simulink model "massbalancer3"  (R2024a)
settings: Solver=ode45  StartTime=0.0  StopTime=300  MaxStep=0.5  RelTol=1e-3
libraries: matrix_library x29, sharedutil x3, sharedtransform x2, dspinverses x1, aerolibutil x1
(part 3 of 3)

== system massbalancer3/TNet/TBalances/Term2/Subsystem1 ==
  R_0 : Inport
  Reshape : Reshape  OutputDimensionality=Column vector (2-D)  OutputDimensions=[1,3]
  Selector : Selector  InputPortWidth=9  IndexOptions=Index vector (dialog)  Indices=[1]  OutputSizes=1
  Selector1 : Selector  InputPortWidth=9  IndexOptions=Index vector (dialog)  Indices=[2]  OutputSizes=1
  Selector2 : Selector  InputPortWidth=9  IndexOptions=Index vector (dialog)  Indices=[3]  OutputSizes=1
  Selector3 : Selector  InputPortWidth=9  IndexOptions=Index vector (dialog)  Indices=[4]  OutputSizes=1
  Selector4 : Selector  InputPortWidth=9  IndexOptions=Index vector (dialog)  Indices=[5]  OutputSizes=1
  Selector5 : Selector  InputPortWidth=9  IndexOptions=Index vector (dialog)  Indices=[6]  OutputSizes=1
  Selector6 : Selector  InputPortWidth=9  IndexOptions=Index vector (dialog)  Indices=[7]  OutputSizes=1
  Selector7 : Selector  InputPortWidth=9  IndexOptions=Index vector (dialog)  Indices=[8]  OutputSizes=1
  Selector8 : Selector  InputPortWidth=9  IndexOptions=Index vector (dialog)  Indices=[9]  OutputSizes=1
  Vector Concatenate : Concatenate  NumInputs=3  Mode=Multidimensional array
  Vector Concatenate1 : Concatenate  NumInputs=3  Mode=Multidimensional array
  Vector Concatenate2 : Concatenate  NumInputs=3  Mode=Multidimensional array
  Out1 : Outport
  Out2 : Outport  Port=2
  Out3 : Outport  Port=3
  wires:
  Selector3/1 -> Vector Concatenate1/1
  Selector1/1 -> Vector Concatenate/2
  Vector Concatenate1/1 -> Out2/1
  Vector Concatenate2/1 -> Out3/1
  Selector7/1 -> Vector Concatenate2/2
  Selector5/1 -> Vector Concatenate1/3
  Selector/1 -> Vector Concatenate/1
  Reshape/1 -> Selector/1, Selector1/1, Selector2/1, Selector3/1, Selector4/1, Selector5/1, Selector6/1, Selector7/1, Selector8/1
  R_0/1 -> Reshape/1
  Selector6/1 -> Vector Concatenate2/1
  Selector4/1 -> Vector Concatenate1/2
  Selector8/1 -> Vector Concatenate2/3
  Vector Concatenate/1 -> Out1/1
  Selector2/1 -> Vector Concatenate/3

== system massbalancer3/TNet/TBalances/Term2/Subsystem3 ==
  R_0 : Inport
  Reshape : Reshape  OutputDimensionality=Column vector (2-D)  OutputDimensions=[1,3]
  Selector : Selector  InputPortWidth=9  IndexOptions=Index vector (dialog)  Indices=[1]  OutputSizes=1
  Selector1 : Selector  InputPortWidth=9  IndexOptions=Index vector (dialog)  Indices=[2]  OutputSizes=1
  Selector2 : Selector  InputPortWidth=9  IndexOptions=Index vector (dialog)  Indices=[3]  OutputSizes=1
  Selector3 : Selector  InputPortWidth=9  IndexOptions=Index vector (dialog)  Indices=[4]  OutputSizes=1
  Selector4 : Selector  InputPortWidth=9  IndexOptions=Index vector (dialog)  Indices=[5]  OutputSizes=1
  Selector5 : Selector  InputPortWidth=9  IndexOptions=Index vector (dialog)  Indices=[6]  OutputSizes=1
  Selector6 : Selector  InputPortWidth=9  IndexOptions=Index vector (dialog)  Indices=[7]  OutputSizes=1
  Selector7 : Selector  InputPortWidth=9  IndexOptions=Index vector (dialog)  Indices=[8]  OutputSizes=1
  Selector8 : Selector  InputPortWidth=9  IndexOptions=Index vector (dialog)  Indices=[9]  OutputSizes=1
  Vector Concatenate : Concatenate  NumInputs=3  Mode=Multidimensional array
  Vector Concatenate1 : Concatenate  NumInputs=3  Mode=Multidimensional array
  Vector Concatenate2 : Concatenate  NumInputs=3  Mode=Multidimensional array
  Out1 : Outport
  Out2 : Outport  Port=2
  Out3 : Outport  Port=3
  wires:
  Selector2/1 -> Vector Concatenate/3
  Vector Concatenate/1 -> Out1/1
  Selector8/1 -> Vector Concatenate2/3
  Selector4/1 -> Vector Concatenate1/2
  Selector6/1 -> Vector Concatenate2/1
  R_0/1 -> Reshape/1
  Reshape/1 -> Selector8/1, Selector7/1, Selector6/1, Selector5/1, Selector4/1, Selector3/1, Selector2/1, Selector1/1, Selector/1
  Selector/1 -> Vector Concatenate/1
  Selector5/1 -> Vector Concatenate1/3
  Selector7/1 -> Vector Concatenate2/2
  Vector Concatenate2/1 -> Out3/1
  Vector Concatenate1/1 -> Out2/1
  Selector1/1 -> Vector Concatenate/2
  Selector3/1 -> Vector Concatenate1/1

== system massbalancer3/TNet/TBalances/Term2/X ==
  R-0 : Inport
  Ddot : Inport  Port=2
  s : Inport  Port=3
  Wb : Inport  Port=4
  Cross Product : matrix_library/Cross Product
  Cross Product1 : matrix_library/Cross Product
  Product : Product
  Output : Outport
  wires:
  Cross Product1/1 -> Output/1
  s/1 -> Product/1
  Ddot/1 -> Product/2
  Product/1 -> Cross Product/2
  Wb/1 -> Cross Product/1
  R-0/1 -> Cross Product1/1
  Cross Product/1 -> Cross Product1/2

== system massbalancer3/TNet/TBalances/Term2/Y ==
  R0 : Inport
  ddot : Inport  Port=2
  s : Inport  Port=3
  Wb : Inport  Port=4
  Cross Product : matrix_library/Cross Product
  Cross Product1 : matrix_library/Cross Product
  Product : Product
  Output : Outport
  wires:
  s/1 -> Product/1
  Product/1 -> Cross Product/2
  R0/1 -> Cross Product1/1
  Cross Product/1 -> Cross Product1/2
  ddot/1 -> Product/2
  Wb/1 -> Cross Product/1
  Cross Product1/1 -> Output/1

== system massbalancer3/TNet/TBalances/Term2/Z ==
  ddot : Inport
  R0 : Inport  Port=2
  s : Inport  Port=3
  Wb : Inport  Port=4
  Cross Product : matrix_library/Cross Product
  Cross Product1 : matrix_library/Cross Product
  Product : Product
  Output1 : Outport
  wires:
  s/1 -> Product/1
  Product/1 -> Cross Product/2
  R0/1 -> Cross Product1/1
  Cross Product/1 -> Cross Product1/2
  ddot/1 -> Product/2
  Wb/1 -> Cross Product/1
  Cross Product1/1 -> Output1/1

== system massbalancer3/TNet/TBalances/Term3/Subsystem1 ==
  R_0 : Inport
  Reshape : Reshape  OutputDimensionality=Column vector (2-D)  OutputDimensions=[1,3]
  Selector : Selector  InputPortWidth=9  IndexOptions=Index vector (dialog)  Indices=[1]  OutputSizes=1
  Selector1 : Selector  InputPortWidth=9  IndexOptions=Index vector (dialog)  Indices=[2]  OutputSizes=1
  Selector2 : Selector  InputPortWidth=9  IndexOptions=Index vector (dialog)  Indices=[3]  OutputSizes=1
  Selector3 : Selector  InputPortWidth=9  IndexOptions=Index vector (dialog)  Indices=[4]  OutputSizes=1
  Selector4 : Selector  InputPortWidth=9  IndexOptions=Index vector (dialog)  Indices=[5]  OutputSizes=1
  Selector5 : Selector  InputPortWidth=9  IndexOptions=Index vector (dialog)  Indices=[6]  OutputSizes=1
  Selector6 : Selector  InputPortWidth=9  IndexOptions=Index vector (dialog)  Indices=[7]  OutputSizes=1
  Selector7 : Selector  InputPortWidth=9  IndexOptions=Index vector (dialog)  Indices=[8]  OutputSizes=1
  Selector8 : Selector  InputPortWidth=9  IndexOptions=Index vector (dialog)  Indices=[9]  OutputSizes=1
  Vector Concatenate : Concatenate  NumInputs=3  Mode=Multidimensional array
  Vector Concatenate1 : Concatenate  NumInputs=3  Mode=Multidimensional array
  Vector Concatenate2 : Concatenate  NumInputs=3  Mode=Multidimensional array
  Out1 : Outport
  Out2 : Outport  Port=2
  Out3 : Outport  Port=3
  wires:
  Selector3/1 -> Vector Concatenate1/1
  Selector1/1 -> Vector Concatenate/2
  Vector Concatenate1/1 -> Out2/1
  Vector Concatenate2/1 -> Out3/1
  Selector7/1 -> Vector Concatenate2/2
  Selector5/1 -> Vector Concatenate1/3
  Selector/1 -> Vector Concatenate/1
  Reshape/1 -> Selector/1, Selector1/1, Selector2/1, Selector3/1, Selector4/1, Selector5/1, Selector6/1, Selector7/1, Selector8/1
  R_0/1 -> Reshape/1
  Selector6/1 -> Vector Concatenate2/1
  Selector4/1 -> Vector Concatenate1/2
  Selector8/1 -> Vector Concatenate2/3
  Vector Concatenate/1 -> Out1/1
  Selector2/1 -> Vector Concatenate/3

== system massbalancer3/TNet/TBalances/Term3/Subsystem3 ==
  R_0 : Inport
  Reshape : Reshape  OutputDimensionality=Column vector (2-D)  OutputDimensions=[1,3]
  Selector : Selector  InputPortWidth=9  IndexOptions=Index vector (dialog)  Indices=[1]  OutputSizes=1
  Selector1 : Selector  InputPortWidth=9  IndexOptions=Index vector (dialog)  Indices=[2]  OutputSizes=1
  Selector2 : Selector  InputPortWidth=9  IndexOptions=Index vector (dialog)  Indices=[3]  OutputSizes=1
  Selector3 : Selector  InputPortWidth=9  IndexOptions=Index vector (dialog)  Indices=[4]  OutputSizes=1
  Selector4 : Selector  InputPortWidth=9  IndexOptions=Index vector (dialog)  Indices=[5]  OutputSizes=1
  Selector5 : Selector  InputPortWidth=9  IndexOptions=Index vector (dialog)  Indices=[6]  OutputSizes=1
  Selector6 : Selector  InputPortWidth=9  IndexOptions=Index vector (dialog)  Indices=[7]  OutputSizes=1
  Selector7 : Selector  InputPortWidth=9  IndexOptions=Index vector (dialog)  Indices=[8]  OutputSizes=1
  Selector8 : Selector  InputPortWidth=9  IndexOptions=Index vector (dialog)  Indices=[9]  OutputSizes=1
  Vector Concatenate : Concatenate  NumInputs=3  Mode=Multidimensional array
  Vector Concatenate1 : Concatenate  NumInputs=3  Mode=Multidimensional array
  Vector Concatenate2 : Concatenate  NumInputs=3  Mode=Multidimensional array
  Out1 : Outport
  Out2 : Outport  Port=2
  Out3 : Outport  Port=3
  wires:
  Selector2/1 -> Vector Concatenate/3
  Vector Concatenate/1 -> Out1/1
  Selector8/1 -> Vector Concatenate2/3
  Selector4/1 -> Vector Concatenate1/2
  Selector6/1 -> Vector Concatenate2/1
  R_0/1 -> Reshape/1
  Reshape/1 -> Selector8/1, Selector7/1, Selector6/1, Selector5/1, Selector4/1, Selector3/1, Selector2/1, Selector1/1, Selector/1
  Selector/1 -> Vector Concatenate/1
  Selector5/1 -> Vector Concatenate1/3
  Selector7/1 -> Vector Concatenate2/2
  Vector Concatenate2/1 -> Out3/1
  Vector Concatenate1/1 -> Out2/1
  Selector1/1 -> Vector Concatenate/2
  Selector3/1 -> Vector Concatenate1/1

== system massbalancer3/TNet/TBalances/Term3/X ==
  ddoubledot : Inport
  s : Inport  Port=2
  r : Inport  Port=3
  Cross Product : matrix_library/Cross Product
  Product : Product
  y : Outport
  wires:
  Cross Product/1 -> y/1
  ddoubledot/1 -> Product/1
  Product/1 -> Cross Product/2
  r/1 -> Cross Product/1
  s/1 -> Product/2

== system massbalancer3/TNet/TBalances/Term3/Y ==
  ddoubledot : Inport
  s : Inport  Port=2
  r : Inport  Port=3
  Cross Product : matrix_library/Cross Product
  Product : Product
  y : Outport
  wires:
  Cross Product/1 -> y/1
  ddoubledot/1 -> Product/1
  Product/1 -> Cross Product/2
  r/1 -> Cross Product/1
  s/1 -> Product/2

== system massbalancer3/TNet/TBalances/Term3/Z ==
  r : Inport
  s : Inport  Port=2
  ddoubledot : Inport  Port=3
  Cross Product : matrix_library/Cross Product
  Display : Display
  Product : Product
  y : Outport
  wires:
  Cross Product/1 -> Display/1, y/1
  ddoubledot/1 -> Product/1
  s/1 -> Product/2
  Product/1 -> Cross Product/2
  r/1 -> Cross Product/1

== system massbalancer3/TNet/Tbalances Init T Gravity /Fgravity/Q(q) rotational form of quaternio ==
  Q_input : Inport
  "(q1,q2,q3,q0) to (q0,q1,q2,q3) " : Subsystem
  Quaternions to Direction Cosine Matrix : sharedtransform/Quaternions to  Direction Cosine Matrix  aMode=aMode
      settings: LibrarySourceBlock=|
      | aerolibtransform2/Quaternions to
      | Direction Cosine Matrix
  Out1 : Outport
  wires:
  "(q1,q2,q3,q0) to (q0,q1,q2,q3) "/1(Output) -> Quaternions to Direction Cosine Matrix/1
  Q_input/1 -> "(q1,q2,q3,q0) to (q0,q1,q2,q3) "/1(Q_input)
  Quaternions to Direction Cosine Matrix/1 -> Out1/1

== system massbalancer3/TNet/Tbalances Init T Gravity /Subsystem/Subsystem2 ==
  In1 : Inport
  Constant : Constant  Value=0  VectorParams1D=off
  Constant1 : Constant  Value=0  VectorParams1D=off
  Constant2 : Constant  Value=0  VectorParams1D=off
  Demux : Demux  Outputs=3
  Gain : Gain  Gain=-1
  Gain1 : Gain  Gain=-1
  Gain2 : Gain  Gain=-1
  Matrix Concatenate : Concatenate  NumInputs=3  Mode=Multidimensional array  ConcatenateDimension=2
  Mux : Mux  Inputs=3
  Mux1 : Mux  Inputs=3
  Mux2 : Mux  Inputs=3
  Output : Outport
  wires:
  Constant/1 -> Mux/1
  Gain2/1 -> Mux2/1
  Gain1/1 -> Mux1/3
  Mux/1 -> Matrix Concatenate/1
  Demux/2 -> Mux/3, Gain2/1
  In1/1 -> Demux/1
  Gain/1 -> Mux/2
  Demux/3 -> Mux1/1, Gain/1
  Mux1/1 -> Matrix Concatenate/2
  Mux2/1 -> Matrix Concatenate/3
  Demux/1 -> Mux2/2, Gain1/1
  Constant1/1 -> Mux1/2
  Constant2/1 -> Mux2/3
  Matrix Concatenate/1 -> Output/1

== system massbalancer3/TNet/Subsystem1/Tbalances Init T Gravity /Fgravity/Q(q) rotational form of quaternio ==
  Q_input : Inport
  "(q1,q2,q3,q0) to (q0,q1,q2,q3) " : Subsystem
  Quaternions to Direction Cosine Matrix : sharedtransform/Quaternions to  Direction Cosine Matrix  aMode=aMode
      settings: LibrarySourceBlock=|
      | aerolibtransform2/Quaternions to
      | Direction Cosine Matrix
  Out1 : Outport
  wires:
  "(q1,q2,q3,q0) to (q0,q1,q2,q3) "/1(Output) -> Quaternions to Direction Cosine Matrix/1
  Q_input/1 -> "(q1,q2,q3,q0) to (q0,q1,q2,q3) "/1(Q_input)
  Quaternions to Direction Cosine Matrix/1 -> Out1/1

== system massbalancer3/TNet/Subsystem1/Term 1/R_I/Subsystem3 ==
  In1 : Inport
  Reshape : Reshape  OutputDimensionality=Column vector (2-D)  OutputDimensions=[1,3]
  Selector : Selector  InputPortWidth=9  IndexOptions=Index vector (dialog)  Indices=[1]  OutputSizes=1
  Selector1 : Selector  InputPortWidth=9  IndexOptions=Index vector (dialog)  Indices=[2]  OutputSizes=1
  Selector2 : Selector  InputPortWidth=9  IndexOptions=Index vector (dialog)  Indices=[3]  OutputSizes=1
  Selector3 : Selector  InputPortWidth=9  IndexOptions=Index vector (dialog)  Indices=[4]  OutputSizes=1
  Selector4 : Selector  InputPortWidth=9  IndexOptions=Index vector (dialog)  Indices=[5]  OutputSizes=1
  Selector5 : Selector  InputPortWidth=9  IndexOptions=Index vector (dialog)  Indices=[6]  OutputSizes=1
  Selector6 : Selector  InputPortWidth=9  IndexOptions=Index vector (dialog)  Indices=[7]  OutputSizes=1
  Selector7 : Selector  InputPortWidth=9  IndexOptions=Index vector (dialog)  Indices=[8]  OutputSizes=1
  Selector8 : Selector  InputPortWidth=9  IndexOptions=Index vector (dialog)  Indices=[9]  OutputSizes=1
  Vector Concatenate : Concatenate  NumInputs=3  Mode=Multidimensional array
  Vector Concatenate1 : Concatenate  NumInputs=3  Mode=Multidimensional array
  Vector Concatenate2 : Concatenate  NumInputs=3  Mode=Multidimensional array
  Out1 : Outport
  Out2 : Outport  Port=2
  Out3 : Outport  Port=3
  wires:
  Selector2/1 -> Vector Concatenate/3
  Vector Concatenate/1 -> Out1/1
  Selector8/1 -> Vector Concatenate2/3
  Selector4/1 -> Vector Concatenate1/2
  Selector6/1 -> Vector Concatenate2/1
  In1/1 -> Reshape/1
  Reshape/1 -> Selector8/1, Selector7/1, Selector6/1, Selector5/1, Selector4/1, Selector3/1, Selector2/1, Selector1/1, Selector/1
  Selector/1 -> Vector Concatenate/1
  Selector5/1 -> Vector Concatenate1/3
  Selector7/1 -> Vector Concatenate2/2
  Vector Concatenate2/1 -> Out3/1
  Vector Concatenate1/1 -> Out2/1
  Selector1/1 -> Vector Concatenate/2
  Selector3/1 -> Vector Concatenate1/1

== system massbalancer3/TNet/Subsystem1/Term 1/R_I/Subsystem4 ==
  In1 : Inport
  Reshape : Reshape  OutputDimensionality=Column vector (2-D)  OutputDimensions=[1,3]
  Selector : Selector  InputPortWidth=9  IndexOptions=Index vector (dialog)  Indices=[1]  OutputSizes=1
  Selector1 : Selector  InputPortWidth=9  IndexOptions=Index vector (dialog)  Indices=[2]  OutputSizes=1
  Selector2 : Selector  InputPortWidth=9  IndexOptions=Index vector (dialog)  Indices=[3]  OutputSizes=1
  Selector3 : Selector  InputPortWidth=9  IndexOptions=Index vector (dialog)  Indices=[4]  OutputSizes=1
  Selector4 : Selector  InputPortWidth=9  IndexOptions=Index vector (dialog)  Indices=[5]  OutputSizes=1
  Selector5 : Selector  InputPortWidth=9  IndexOptions=Index vector (dialog)  Indices=[6]  OutputSizes=1
  Selector6 : Selector  InputPortWidth=9  IndexOptions=Index vector (dialog)  Indices=[7]  OutputSizes=1
  Selector7 : Selector  InputPortWidth=9  IndexOptions=Index vector (dialog)  Indices=[8]  OutputSizes=1
  Selector8 : Selector  InputPortWidth=9  IndexOptions=Index vector (dialog)  Indices=[9]  OutputSizes=1
  Vector Concatenate : Concatenate  NumInputs=3  Mode=Multidimensional array
  Vector Concatenate1 : Concatenate  NumInputs=3  Mode=Multidimensional array
  Vector Concatenate2 : Concatenate  NumInputs=3  Mode=Multidimensional array
  Out1 : Outport
  Out2 : Outport  Port=2
  Out3 : Outport  Port=3
  wires:
  Selector3/1 -> Vector Concatenate1/1
  Selector1/1 -> Vector Concatenate/2
  Vector Concatenate1/1 -> Out2/1
  Vector Concatenate2/1 -> Out3/1
  Selector7/1 -> Vector Concatenate2/2
  Selector5/1 -> Vector Concatenate1/3
  Selector/1 -> Vector Concatenate/1
  Reshape/1 -> Selector/1, Selector1/1, Selector2/1, Selector3/1, Selector4/1, Selector5/1, Selector6/1, Selector7/1, Selector8/1
  In1/1 -> Reshape/1
  Selector6/1 -> Vector Concatenate2/1
  Selector4/1 -> Vector Concatenate1/2
  Selector8/1 -> Vector Concatenate2/3
  Vector Concatenate/1 -> Out1/1
  Selector2/1 -> Vector Concatenate/3

== system massbalancer3/TNet/Subsystem1/Term 1/X/Subsystem ==
  Wb : Inport
  Constant : Constant  Value=0  VectorParams1D=off
  Constant1 : Constant  Value=0  VectorParams1D=off
  Constant2 : Constant  Value=0  VectorParams1D=off
  Demux : Demux  Outputs=3
  Gain : Gain  Gain=-1
  Gain1 : Gain  Gain=-1
  Gain2 : Gain  Gain=-1
  Matrix Concatenate : Concatenate  NumInputs=3  Mode=Multidimensional array  ConcatenateDimension=2
  Mux : Mux  Inputs=3
  Mux1 : Mux  Inputs=3
  Mux2 : Mux  Inputs=3
  Out1 : Outport
  wires:
  Constant/1 -> Mux/1
  Gain2/1 -> Mux2/1
  Gain1/1 -> Mux1/3
  Mux/1 -> Matrix Concatenate/1
  Demux/2 -> Mux/3, Gain2/1
  Wb/1 -> Demux/1
  Gain/1 -> Mux/2
  Demux/3 -> Mux1/1, Gain/1
  Mux1/1 -> Matrix Concatenate/2
  Mux2/1 -> Matrix Concatenate/3
  Demux/1 -> Mux2/2, Gain1/1
  Constant1/1 -> Mux1/2
  Constant2/1 -> Mux2/3
  Matrix Concatenate/1 -> Out1/1

== system massbalancer3/TNet/Subsystem1/Term 1/X/Subsystem1 ==
  In1 : Inport
  Constant : Constant  Value=0  VectorParams1D=off
  Constant1 : Constant  Value=0  VectorParams1D=off
  Constant2 : Constant  Value=0  VectorParams1D=off
  Demux : Demux  Outputs=3
  Gain : Gain  Gain=-1
  Gain1 : Gain  Gain=-1
  Gain2 : Gain  Gain=-1
  Matrix Concatenate : Concatenate  NumInputs=3  Mode=Multidimensional array  ConcatenateDimension=2
  Mux : Mux  Inputs=3
  Mux1 : Mux  Inputs=3
  Mux2 : Mux  Inputs=3
  Out1 : Outport
  wires:
  Constant/1 -> Mux/1
  Gain2/1 -> Mux2/1
  Gain1/1 -> Mux1/3
  Mux/1 -> Matrix Concatenate/1
  Demux/2 -> Mux/3, Gain2/1
  In1/1 -> Demux/1
  Gain/1 -> Mux/2
  Demux/3 -> Mux1/1, Gain/1
  Mux1/1 -> Matrix Concatenate/2
  Mux2/1 -> Matrix Concatenate/3
  Demux/1 -> Mux2/2, Gain1/1
  Constant1/1 -> Mux1/2
  Constant2/1 -> Mux2/3
  Matrix Concatenate/1 -> Out1/1

== system massbalancer3/TNet/Subsystem1/Term 1/Y/Subsystem ==
  In1 : Inport
  Constant : Constant  Value=0  VectorParams1D=off
  Constant1 : Constant  Value=0  VectorParams1D=off
  Constant2 : Constant  Value=0  VectorParams1D=off
  Demux : Demux  Outputs=3
  Gain : Gain  Gain=-1
  Gain1 : Gain  Gain=-1
  Gain2 : Gain  Gain=-1
  Matrix Concatenate : Concatenate  NumInputs=3  Mode=Multidimensional array  ConcatenateDimension=2
  Mux : Mux  Inputs=3
  Mux1 : Mux  Inputs=3
  Mux2 : Mux  Inputs=3
  Out1 : Outport
  wires:
  Constant/1 -> Mux/1
  Gain2/1 -> Mux2/1
  Gain1/1 -> Mux1/3
  Mux/1 -> Matrix Concatenate/1
  Demux/2 -> Mux/3, Gain2/1
  In1/1 -> Demux/1
  Gain/1 -> Mux/2
  Demux/3 -> Mux1/1, Gain/1
  Mux1/1 -> Matrix Concatenate/2
  Mux2/1 -> Matrix Concatenate/3
  Demux/1 -> Mux2/2, Gain1/1
  Constant1/1 -> Mux1/2
  Constant2/1 -> Mux2/3
  Matrix Concatenate/1 -> Out1/1

== system massbalancer3/TNet/Subsystem1/Term 1/Y/Subsystem1 ==
  In1 : Inport
  Constant : Constant  Value=0  VectorParams1D=off
  Constant1 : Constant  Value=0  VectorParams1D=off
  Constant2 : Constant  Value=0  VectorParams1D=off
  Demux : Demux  Outputs=3
  Gain : Gain  Gain=-1
  Gain1 : Gain  Gain=-1
  Gain2 : Gain  Gain=-1
  Matrix Concatenate : Concatenate  NumInputs=3  Mode=Multidimensional array  ConcatenateDimension=2
  Mux : Mux  Inputs=3
  Mux1 : Mux  Inputs=3
  Mux2 : Mux  Inputs=3
  Out1 : Outport
  wires:
  Constant/1 -> Mux/1
  Gain2/1 -> Mux2/1
  Gain1/1 -> Mux1/3
  Mux/1 -> Matrix Concatenate/1
  Demux/2 -> Mux/3, Gain2/1
  In1/1 -> Demux/1
  Gain/1 -> Mux/2
  Demux/3 -> Mux1/1, Gain/1
  Mux1/1 -> Matrix Concatenate/2
  Mux2/1 -> Matrix Concatenate/3
  Demux/1 -> Mux2/2, Gain1/1
  Constant1/1 -> Mux1/2
  Constant2/1 -> Mux2/3
  Matrix Concatenate/1 -> Out1/1

== system massbalancer3/TNet/Subsystem1/Term 1/Z/Subsystem1 ==
  In1 : Inport
  Constant : Constant  Value=0  VectorParams1D=off
  Constant1 : Constant  Value=0  VectorParams1D=off
  Constant2 : Constant  Value=0  VectorParams1D=off
  Demux : Demux  Outputs=3
  Gain : Gain  Gain=-1
  Gain1 : Gain  Gain=-1
  Gain2 : Gain  Gain=-1
  Matrix Concatenate : Concatenate  NumInputs=3  Mode=Multidimensional array  ConcatenateDimension=2
  Mux : Mux  Inputs=3
  Mux1 : Mux  Inputs=3
  Mux2 : Mux  Inputs=3
  Out1 : Outport
  wires:
  Constant/1 -> Mux/1
  Gain2/1 -> Mux2/1
  Gain1/1 -> Mux1/3
  Mux/1 -> Matrix Concatenate/1
  Demux/2 -> Mux/3, Gain2/1
  In1/1 -> Demux/1
  Gain/1 -> Mux/2
  Demux/3 -> Mux1/1, Gain/1
  Mux1/1 -> Matrix Concatenate/2
  Mux2/1 -> Matrix Concatenate/3
  Demux/1 -> Mux2/2, Gain1/1
  Constant1/1 -> Mux1/2
  Constant2/1 -> Mux2/3
  Matrix Concatenate/1 -> Out1/1

== system massbalancer3/TNet/Subsystem1/Term 1/Z/Subsystem2 ==
  In1 : Inport
  Constant : Constant  Value=0  VectorParams1D=off
  Constant1 : Constant  Value=0  VectorParams1D=off
  Constant2 : Constant  Value=0  VectorParams1D=off
  Demux : Demux  Outputs=3
  Gain : Gain  Gain=-1
  Gain1 : Gain  Gain=-1
  Gain2 : Gain  Gain=-1
  Matrix Concatenate : Concatenate  NumInputs=3  Mode=Multidimensional array  ConcatenateDimension=2
  Mux : Mux  Inputs=3
  Mux1 : Mux  Inputs=3
  Mux2 : Mux  Inputs=3
  Out1 : Outport
  wires:
  Matrix Concatenate/1 -> Out1/1
  Constant2/1 -> Mux2/3
  Constant1/1 -> Mux1/2
  Demux/1 -> Gain1/1, Mux2/2
  Mux2/1 -> Matrix Concatenate/3
  Mux1/1 -> Matrix Concatenate/2
  Demux/3 -> Gain/1, Mux1/1
  Gain/1 -> Mux/2
  In1/1 -> Demux/1
  Demux/2 -> Gain2/1, Mux/3
  Mux/1 -> Matrix Concatenate/1
  Gain1/1 -> Mux1/3
  Gain2/1 -> Mux2/1
  Constant/1 -> Mux/1

== system massbalancer3/TNet/Subsystem1/Term2/R_I/Subsystem3 ==
  In1 : Inport
  Reshape : Reshape  OutputDimensionality=Column vector (2-D)  OutputDimensions=[1,3]
  Selector : Selector  InputPortWidth=9  IndexOptions=Index vector (dialog)  Indices=[1]  OutputSizes=1
  Selector1 : Selector  InputPortWidth=9  IndexOptions=Index vector (dialog)  Indices=[2]  OutputSizes=1
  Selector2 : Selector  InputPortWidth=9  IndexOptions=Index vector (dialog)  Indices=[3]  OutputSizes=1
  Selector3 : Selector  InputPortWidth=9  IndexOptions=Index vector (dialog)  Indices=[4]  OutputSizes=1
  Selector4 : Selector  InputPortWidth=9  IndexOptions=Index vector (dialog)  Indices=[5]  OutputSizes=1
  Selector5 : Selector  InputPortWidth=9  IndexOptions=Index vector (dialog)  Indices=[6]  OutputSizes=1
  Selector6 : Selector  InputPortWidth=9  IndexOptions=Index vector (dialog)  Indices=[7]  OutputSizes=1
  Selector7 : Selector  InputPortWidth=9  IndexOptions=Index vector (dialog)  Indices=[8]  OutputSizes=1
  Selector8 : Selector  InputPortWidth=9  IndexOptions=Index vector (dialog)  Indices=[9]  OutputSizes=1
  Vector Concatenate : Concatenate  NumInputs=3  Mode=Multidimensional array
  Vector Concatenate1 : Concatenate  NumInputs=3  Mode=Multidimensional array
  Vector Concatenate2 : Concatenate  NumInputs=3  Mode=Multidimensional array
  Out1 : Outport
  Out2 : Outport  Port=2
  Out3 : Outport  Port=3
  wires:
  Selector2/1 -> Vector Concatenate/3
  Vector Concatenate/1 -> Out1/1
  Selector8/1 -> Vector Concatenate2/3
  Selector4/1 -> Vector Concatenate1/2
  Selector6/1 -> Vector Concatenate2/1
  In1/1 -> Reshape/1
  Reshape/1 -> Selector8/1, Selector7/1, Selector6/1, Selector5/1, Selector4/1, Selector3/1, Selector2/1, Selector1/1, Selector/1
  Selector/1 -> Vector Concatenate/1
  Selector5/1 -> Vector Concatenate1/3
  Selector7/1 -> Vector Concatenate2/2
  Vector Concatenate2/1 -> Out3/1
  Vector Concatenate1/1 -> Out2/1
  Selector1/1 -> Vector Concatenate/2
  Selector3/1 -> Vector Concatenate1/1

== system massbalancer3/TNet/Subsystem1/Term2/R_I/Subsystem4 ==
  In1 : Inport
  Reshape : Reshape  OutputDimensionality=Column vector (2-D)  OutputDimensions=[1,3]
  Selector : Selector  InputPortWidth=9  IndexOptions=Index vector (dialog)  Indices=[1]  OutputSizes=1
  Selector1 : Selector  InputPortWidth=9  IndexOptions=Index vector (dialog)  Indices=[2]  OutputSizes=1
  Selector2 : Selector  InputPortWidth=9  IndexOptions=Index vector (dialog)  Indices=[3]  OutputSizes=1
  Selector3 : Selector  InputPortWidth=9  IndexOptions=Index vector (dialog)  Indices=[4]  OutputSizes=1
  Selector4 : Selector  InputPortWidth=9  IndexOptions=Index vector (dialog)  Indices=[5]  OutputSizes=1
  Selector5 : Selector  InputPortWidth=9  IndexOptions=Index vector (dialog)  Indices=[6]  OutputSizes=1
  Selector6 : Selector  InputPortWidth=9  IndexOptions=Index vector (dialog)  Indices=[7]  OutputSizes=1
  Selector7 : Selector  InputPortWidth=9  IndexOptions=Index vector (dialog)  Indices=[8]  OutputSizes=1
  Selector8 : Selector  InputPortWidth=9  IndexOptions=Index vector (dialog)  Indices=[9]  OutputSizes=1
  Vector Concatenate : Concatenate  NumInputs=3  Mode=Multidimensional array
  Vector Concatenate1 : Concatenate  NumInputs=3  Mode=Multidimensional array
  Vector Concatenate2 : Concatenate  NumInputs=3  Mode=Multidimensional array
  Out1 : Outport
  Out2 : Outport  Port=2
  Out3 : Outport  Port=3
  wires:
  Selector3/1 -> Vector Concatenate1/1
  Selector1/1 -> Vector Concatenate/2
  Vector Concatenate1/1 -> Out2/1
  Vector Concatenate2/1 -> Out3/1
  Selector7/1 -> Vector Concatenate2/2
  Selector5/1 -> Vector Concatenate1/3
  Selector/1 -> Vector Concatenate/1
  Reshape/1 -> Selector/1, Selector1/1, Selector2/1, Selector3/1, Selector4/1, Selector5/1, Selector6/1, Selector7/1, Selector8/1
  In1/1 -> Reshape/1
  Selector6/1 -> Vector Concatenate2/1
  Selector4/1 -> Vector Concatenate1/2
  Selector8/1 -> Vector Concatenate2/3
  Vector Concatenate/1 -> Out1/1
  Selector2/1 -> Vector Concatenate/3

== system massbalancer3/TNet/Tbalances Init T Gravity /Fgravity/Q(q) rotational form of quaternio/(q1,q2,q3,q0) to (q0,q1,q2,q3)  ==
  Q_input : Inport
  Quaternion Normalize : sharedutil/Quaternion Normalize  aMode=aMode
  Vector Concatenate : Concatenate
  e_q_vect1 : Selector  InputPortWidth=4  IndexOptions=Index vector (dialog)  Indices=[1 2 3]  OutputSizes=1
  e_q_vect2 : Selector  InputPortWidth=4  IndexOptions=Index vector (dialog)  Indices=[4]  OutputSizes=1
  Output : Outport
  wires:
  Q_input/1 -> e_q_vect2/1, e_q_vect1/1
  e_q_vect2/1 -> Vector Concatenate/1
  e_q_vect1/1 -> Vector Concatenate/2
  Vector Concatenate/1 -> Quaternion Normalize/1
  Quaternion Normalize/1 -> Output/1

== system massbalancer3/TNet/Subsystem1/Tbalances Init T Gravity /Fgravity/Q(q) rotational form of quaternio/(q1,q2,q3,q0) to (q0,q1,q2,q3)  ==
  Q_input : Inport
  Quaternion Normalize : sharedutil/Quaternion Normalize  aMode=aMode
  Vector Concatenate : Concatenate
  e_q_vect1 : Selector  InputPortWidth=4  IndexOptions=Index vector (dialog)  Indices=[1 2 3]  OutputSizes=1
  e_q_vect2 : Selector  InputPortWidth=4  IndexOptions=Index vector (dialog)  Indices=[4]  OutputSizes=1
  Output : Outport
  wires:
  Q_input/1 -> e_q_vect2/1, e_q_vect1/1
  e_q_vect2/1 -> Vector Concatenate/1
  e_q_vect1/1 -> Vector Concatenate/2
  Vector Concatenate/1 -> Quaternion Normalize/1
  Quaternion Normalize/1 -> Output/1
